simulink model "l1_lqr"  (R2025b)
settings: Solver=VariableStepAuto  StartTime=0.0  StopTime=10.0  RelTol=1e-3
undefined symbols (not defined in the file or in its folder): P
settings Model: Creator=eshikapathak  LastModifiedBy=eshikapathak

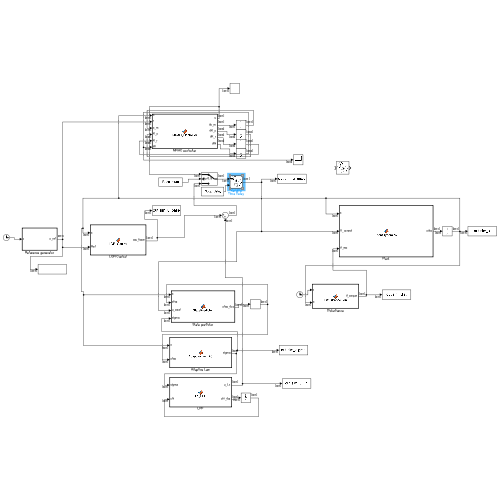
[thumbnail: Simulink's stored preview of the top-level diagram]
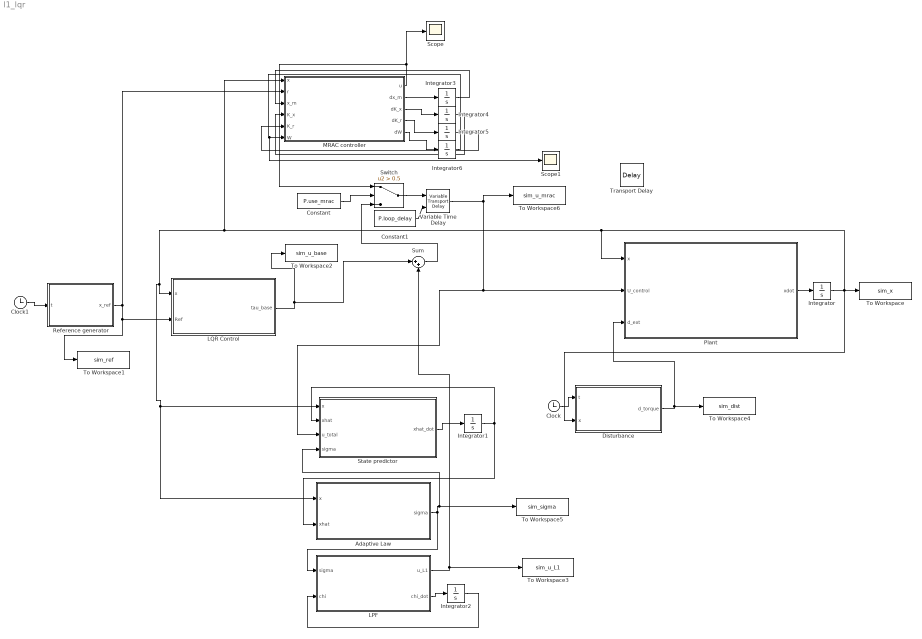
== system l1_lqr ==
  Adaptive Law : MATLAB Function  TreatAsAtomicUnit=on
  Clock : Clock
  Clock1 : Clock
  Constant : Constant  Value=P.use_mrac
  Constant1 : Constant  Value=P.loop_delay
  Disturbance : MATLAB Function  TreatAsAtomicUnit=on
  Integrator{,1..3} (4 alike) : Integrator
  Integrator4 : Integrator  InitialCondition=zeros(3,6)
  Integrator5 : Integrator  InitialCondition=zeros(3,6)
  Integrator6 : Integrator  InitialCondition=zeros(6,3)
  LPF : MATLAB Function  TreatAsAtomicUnit=on
  LQR Control : MATLAB Function  TreatAsAtomicUnit=on
  MRAC controller : MATLAB Function  TreatAsAtomicUnit=on
  Plant : MATLAB Function  TreatAsAtomicUnit=on
  Reference generator : MATLAB Function  TreatAsAtomicUnit=on
  Scope : Scope
      settings: ActiveDisplayYMinimum=-0.18899254495545503  ActiveDisplayYMaximum=0.88826024956797955
  Scope1 : Scope
      settings: ActiveDisplayYMinimum=-17.081145138179366  ActiveDisplayYMaximum=47.040865807014455
  State predictor : MATLAB Function  TreatAsAtomicUnit=on
  Sum : Sum  Inputs=|++
  Switch : Switch  Criteria=u2 > Threshold  Threshold=0.5  SaturateOnIntegerOverflow=off  InputSameDT=off
  To Workspace : ToWorkspace  VariableName=sim_x  SaveFormat=Timeseries  SampleTime=-1
  To Workspace1 : ToWorkspace  VariableName=sim_ref  SaveFormat=Timeseries  SampleTime=-1
  To Workspace2 : ToWorkspace  VariableName=sim_u_base  SaveFormat=Timeseries  SampleTime=-1
  To Workspace3 : ToWorkspace  VariableName=sim_u_L1  SaveFormat=Timeseries  SampleTime=-1
  To Workspace4 : ToWorkspace  VariableName=sim_dist  SaveFormat=Timeseries  SampleTime=-1
  To Workspace5 : ToWorkspace  VariableName=sim_sigma  SaveFormat=Timeseries  SampleTime=-1
  To Workspace6 : ToWorkspace  VariableName=sim_u_mrac  SaveFormat=Timeseries  SampleTime=-1
  Transport Delay : TransportDelay  DelayTime=P.loop_delay  BufferSize=10000000
  Variable Time Delay : VariableTransportDelay  MaximumDelay=10  MaximumPoints=1000000  ZeroDelay=on
  wires:
  Plant/1(xdot) -> Integrator/1
  Integrator/1 -> Disturbance/2(x), To Workspace/1, Plant/1(x), MRAC controller/1(x), LQR Control/1(x), Adaptive Law/1(x), State predictor/1(x)
  Reference generator/1(x_ref) -> LQR Control/2(Ref), To Workspace1/1, MRAC controller/2(r)
  Clock/1 -> Disturbance/1(t)
  Clock1/1 -> Reference generator/1(t)
  LQR Control/1(tau_base) -> To Workspace2/1, Sum/1
  LPF/1(u_L1) -> To Workspace3/1, Sum/2
  State predictor/1(xhat_dot) -> Integrator1/1
  Integrator1/1 -> Adaptive Law/2(xhat), State predictor/2(xhat)
  Adaptive Law/1(sigma) -> To Workspace5/1, State predictor/4(sigma), LPF/1(sigma)
  LPF/2(chi_dot) -> Integrator2/1
  Integrator2/1 -> LPF/2(chi)
  Variable Time Delay/1 -> To Workspace6/1, State predictor/3(u_total), Plant/2(U_control)
  Disturbance/1(d_torque) -> To Workspace4/1, Plant/3(d_ext)
  Switch/1 -> Variable Time Delay/1
  MRAC controller/2(dx_m) -> Integrator3/1
  MRAC controller/3(dK_x) -> Integrator4/1
  MRAC controller/4(dK_r) -> Integrator5/1
  Integrator3/1 -> MRAC controller/3(x_m)
  Integrator4/1 -> MRAC controller/4(K_x)
  Integrator5/1 -> MRAC controller/5(K_r)
  MRAC controller/1(u) -> Scope/1, Switch/1
  Sum/1 -> Switch/3
  Constant/1 -> Switch/2
  MRAC controller/5(dW) -> Integrator6/1
  Integrator6/1 -> Scope1/1, MRAC controller/6(W)
  Constant1/1 -> Variable Time Delay/2

== matlab function l1_lqr/LQR Control ==
  settings: sampleTime=P.Ts/100
  data: x input; tau_base output size=[3 1]; Ref input; P parameter
function tau_base = LQR_Control(x, Ref, P)
    % Standard State Feedback
    error = x - Ref;
    tau_base = -P.K * error;
end

== matlab function l1_lqr/Plant ==
  data: x input; xdot output size=[6 1]; U_control input; d_ext input; P parameter
function xdot = PlantDynamics(x, U_control, d_ext, P)
    % Unpack parameters
    Ix = P.Ix; Iy = P.Iy; Iz = P.Iz; L = P.L;
    
    % States
    % x = [phi, theta, psi, p, q, r]
    p = x(4); q = x(5); r = x(6);
    
    % Total Torque = Control Input + External Disturbance
    % U_control is [U2(Roll), U3(Pitch), U4(Yaw)] 
    % Inputs to this block are TORQUES.
    
    tau_phi   = L * U_control(1) + d_ext(1);
    tau_theta = L * U_control(2) + d_ext(2);
    tau_psi   =     U_control(3) + d_ext(3); 
    
    % Rotational Dynamics (Euler Equations)
    p_dot = q*r*(Iy - Iz)/Ix + (1/Ix) * tau_phi;
    q_dot = p*r*(Iz - Ix)/Iy + (1/Iy) * tau_theta;
    r_dot = p*q*(Ix - Iy)/Iz + (1/Iz) * tau_psi;
    
    % Kinematics 
    phi_dot   = p;
    theta_dot = q;
    psi_dot   = r;
    
    xdot = [phi_dot; theta_dot; psi_dot; p_dot; q_dot; r_dot];
end

== matlab function l1_lqr/State predictor ==
  data: x input; xhat_dot output size=[6 1]; xhat input; u_total input; sigma input; P parameter
% function xhat_dot = StatePredictor(x, xhat, u_total, sigma, P)
function xhat_dot = StatePredictor(x, xhat, u_total, sigma, P)
    % Unpack sigma into Matched (m) and Unmatched (um)
    sigma_m  = sigma(1:3);
    sigma_um = sigma(4:6);

    xt = xhat - x;

    % Predictor Dynamics
    % xhat_dot = A*xhat + Bm*(u + sigma_m) + Bum*sigma_um + Ae*xt
    xhat_dot = P.A_true * x ...
             + P.Bm * (u_total + sigma_m) ...
             + P.Bum * sigma_um ...
             + P.Ae * xt;
end


%%  Nonlinear State Predictor for L1 Adaptive Control
% function xhat_dot = StatePredictor(x, xhat, u_total, sigma, P)
%     % Nonlinear State Predictor for L1 Adaptive Control
%     % Dynamics: xhat_dot = f(x, u) + Bm*sigma_m + Bum*sigma_um + Ae*xt
% 
%     % 1. Unpack Parameters
%     Ix = P.Ix; Iy = P.Iy; Iz = P.Iz; L = P.L;
% 
%     % 2. Unpack Estimated States (from xhat, NOT x)
%     % xhat = [phi, theta, psi, p, q, r]
%     p = x(4); 
%     q = x(5); 
%     r = x(6);
% 
%     % 3. Unpack Control Inputs (Forces/Torque)
%     % u_total = [RollForce, PitchForce, YawTorque]
%     U_roll  = u_total(1);
%     U_pitch = u_total(2);
%     U_yaw   = u_total(3);
% 
%     % 4. Calculate Nominal Nonlinear Dynamics: f(xhat, u)
%     % Kinematics 
%     phi_dot   = p;
%     theta_dot = q;
%     psi_dot   = r;
% 
%     % Rotational Dynamics (Nonlinear Euler Equations)
%     % Note: We apply the same physics scaling (L/I) as the Plant
%     p_dot = ( (Iy - Iz) * q * r + L * U_roll  ) / Ix;
%     q_dot = ( (Iz - Ix) * p * r + L * U_pitch ) / Iy;
%     r_dot = ( (Ix - Iy) * p * q +     U_yaw   ) / Iz;
% 
%     f_x_u = [phi_dot; theta_dot; psi_dot; p_dot; q_dot; r_dot];
% 
%     % 5. Adaptive Augmentation
%     % sigma_m (Matched) affects accelerations
%     % sigma_um (Unmatched) affects kinematics
%     sigma_m  = sigma(1:3);
%     sigma_um = sigma(4:6);
% 
%     % Map Sigma to State Space
%     % P.Bm already contains the 1/J and L/J scaling for the matched uncertainty
%     adaptive_term = P.Bm * sigma_m + P.Bum * sigma_um;
% 
%     % 6. Error Dynamics Injection (Stabilizing term)
%     xt = xhat - x;
%     error_correction = P.Ae * xt;
% 
%     % 7. Final Predictor Derivative
%     xhat_dot = f_x_u + adaptive_term + error_correction;
% end

== matlab function l1_lqr/Adaptive Law ==
  settings: updateMethod=DISCRETE  sampleTime=P.Ts
  data: x input; sigma output size=[6 1]; xhat input; P parameter
function sigma = AdaptiveLaw_PC(x, xhat, P)
    % Define persistent variables to hold sigma for the interval
    % Note: Sampling property of this block is set to discrete with sample time as P.Ts
    persistent sigma_hold
    if isempty(sigma_hold)
        sigma_hold = zeros(6,1);
    end
    
    % Error
    xt = xhat - x;
    
    % Calculations (Closed Form Piecewise Constant)
    % Phi = Ae^-1 * (exp(Ae*Ts) - I)
    % We calculate this dynamically or pass it in. 
    % For efficiency, perform this only once or pass pre-calcs in P.
    
    Phi = P.Ae \ (expm(P.Ae*P.Ts) - eye(6));
    E   = expm(P.Ae*P.Ts);
    
    % z = Phi^-1 * exp(Ae*Ts) * xt(k)
    z = Phi \ (E * xt);
    
    % Bbar * sigma = -z
    % Bbar is square (6x6) because it is [Bm Bum]
    Bbar = [P.Bm, P.Bum];
    
    sigma_new = -(Bbar \ z);
    
    sigma = sigma_new;
end

== matlab function l1_lqr/LPF ==
  data: sigma input; u_L1 output size=[3 1]; chi input; chi_dot output size=[3 1]; P parameter
function [u_L1, chi_dot] = L1_LPF(sigma, chi, P)
    % 1. Extract Matched Uncertainty
    % The LPF only filters the matched component (first 3 elements)
    sigma_m = sigma(1:3);
    
    % 2. Filter Dynamics (State Space)
    % chi_dot = Alpf * chi + Blpf * sigma_m
    chi_dot = P.Alpf * chi + P.Blpf * sigma_m;
    
    % 3. Calculate Control Signal
    % u_L1 = - (Clpf * chi) 
    % We apply the negative sign here to cancel the disturbance.
    % (Dlpf is zero in this design, so we skip it)
    
    u_L1 = -(P.Clpf * chi);
end

== matlab function l1_lqr/Reference generator ==
  data: t input; x_ref output size=[6 1]; P parameter
function x_ref = ReferenceGen(t, P)
    % P.ref_type: 0 = Step, 1 = Sine
    
    ref_roll = 0;
    
    if P.ref_type == 0
        % --- STEP REFERENCE ---
        if t >= P.ref_start
            ref_roll = P.ref_amp;
        end
    else
        % --- SINE REFERENCE ---
        % Amplitude * sin(freq * t)
        % Using fixed 0.5 rad/s freq for testing
        ref_roll = P.ref_amp * sin(1.0 * t); 
    end
    
    % Output: [phi; theta; psi; p; q; r]
    x_ref = [ref_roll; 0; 0; 0; 0; 0];
end

== matlab function l1_lqr/Disturbance ==
  data: t input; x input; d_torque output size=[3 1]; P parameter
function d_torque = DisturbanceGen(t, x, P)
    % Generates disturbance torques (Nm) based on P.dist_type
    % Accepts state 'x' for state-dependent disturbances
    % P.dist_type: 
    %   0 = Single Sine
    %   1 = Sum of High Freq Sines
    %   2 = Triangle / Sawtooth
    %   3 = State-Dependent (Nonlinear)
    
    if isfield(P, 'dist_type')
        type = P.dist_type;
    else
        type = 0;
    end
    
    d_val = 0;

    if type == 0
        % Single Sine
        d_phi   = P.dist_amp(1) * sin(P.dist_freq(1) * t);
        d_theta = P.dist_amp(2) * sin(P.dist_freq(2) * t);
        d_psi   = P.dist_amp(3) * sin(P.dist_freq(3) * t);
        d_torque = [d_phi; d_theta; d_psi];
        return;
        
    elseif type == 1
        % Sum of Sines
        amp = P.dist_amp(1);
        d_val = 0.5 * amp * (sin(20*t) + sin(30*t) + sin(50*t));
        
    elseif type == 2
        % Triangle Wave
        freq = 2.0; amp = P.dist_amp(1);
        T = 2*pi/freq; norm_t = t/T;
        wave = 2 * abs(2 * (norm_t - floor(norm_t + 0.5))) - 1;
        d_val = amp * wave;
        
    elseif type == 3
        % --- STATE DEPENDENT (NONLINEAR) ---
        % d(x) = A * sin(3*phi) * p
        phi = x(1);
        p   = x(4);
        amp = P.dist_amp(1);
        
        d_val = amp * sin(3*phi) * p;
    end
    
    d_torque = [d_val; 0; 0]; 
end

== matlab function l1_lqr/MRAC controller ==
  data: x input; u output size=[3 1]; r input; x_m input size=[6 1]; K_x input; K_r input; W input; dx_m output; dK_x output size=[3 6]; dK_r output size=[3 6]; P parameter; dW output size=[6 3]
function [u, dx_m, dK_x, dK_r, dW] = MRAC_Controller(x, r, x_m, K_x, K_r, W, P)
    % --- 1. UNPACK PARAMETERS ---
    Am = P.MRAC.Am;
    Bm = P.MRAC.Bm;
    Gam_x = P.MRAC.Gam_x;
    Gam_r = P.MRAC.Gam_r;
    Gam_w = P.MRAC.Gam_w; 
    P_lyap = P.MRAC.P_lyap;
    B = P.Bm; 
    
    % Bounds for Projection (from P struct)
    th_x_max = P.MRAC.theta_x_max;
    th_r_max = P.MRAC.theta_r_max;
    th_w_max = P.MRAC.theta_w_max;
    
    % --- 2. BASIS FUNCTIONS (Phi) ---
    p = x(4); q = x(5); rr = x(6); 
    Phi = [tanh(q*rr); tanh(p*rr); tanh(p*q); tanh(p); tanh(q); tanh(rr)];
           
    % --- 3. DYNAMICS & ERROR ---
    dx_m = Am * x_m + Bm * r;
    e = x - x_m;
    
    % --- 4. ADAPTATION DRIVE ---
    % Common term: B' * P * e
    drive = B' * P_lyap * e; 
    
    % --- 5. NOMINAL ADAPTIVE LAWS ---
    dK_x_nom = Gam_x * drive * x'; 
    dK_r_nom = -Gam_r * drive * r'; 
    dW_nom   = Gam_w * Phi * drive'; % Note: dW is typically Gamma * Phi * e'PB
    % Dimension check: Phi(6x1) * drive'(1x3) = 6x3. W is 6x3. Correct.
    
    % --- 6. PROJECTION OPERATOR ---
    % Apply projection to keep parameters bounded
    dK_x = Projection(K_x, dK_x_nom, th_x_max);
    dK_r = Projection(K_r, dK_r_nom, th_r_max);
    dW   = Projection(W,   dW_nom,   th_w_max);
    
    % --- 7. CONTROL LAW ---
    % u = -K_x*x + K_r*r - W'*Phi
    u = -K_x * x + K_r * r - W' * Phi;
end

% --- LOCAL HELPER FUNCTION: PROJECTION ---
function dy_proj = Projection(theta, dy, theta_max)
    % Implements Convex Projection Operator 
    % theta: Current parameter value (matrix or vector)
    % dy:    Nominal update rate
    % theta_max: Maximum allowed Frobenius norm
    
    epsilon = 0.1; % Smoothness buffer width
    
    % 1. Calculate Norm squared
    n2 = sum(sum(theta.^2)); % Squared Frobenius Norm
    th_max2 = theta_max^2;
    
    % 2. Convex Function f(theta)
    f = (n2 - th_max2) / (epsilon * th_max2);
    
    % 3. Gradient of f w.r.t theta
    % grad_f = (2 / (epsilon * theta_max^2)) * theta
    % We only need the direction, so we use theta itself for dot product logic
    
    % Check condition: Are we outside bounds AND trying to grow further?
    % Dot product of Gradient and Update Direction:
    grad_dot_dy = sum(sum(theta .* dy)); 
    
    if (f >= 0) && (grad_dot_dy > 0)
        % ACTIVE PROJECTION
        % Subtract the component of dy that points "outward" (normal to boundary)
        
        % Simplified Smooth Projection Formula:
        % dy_proj = dy - ( (grad_f' * dy) / ||grad_f||^2 ) * grad_f * f(theta)
        
        % Calculating terms for matrices:
        grad_f = (2 / (epsilon * th_max2)) * theta;
        grad_norm2 = sum(sum(grad_f.^2));
        grad_dot_dy_val = sum(sum(grad_f .* dy));
        
        % Avoid divide by zero if theta is 0 (shouldn't happen at boundary)
        if grad_norm2 > 1e-10
            subtraction = (grad_f * grad_dot_dy_val / grad_norm2) * min(1, f);
            dy_proj = dy - subtraction;
        else
            dy_proj = dy;
        end
    else
        % NO PROJECTION (Inside bounds or moving inwards)
        dy_proj = dy;
    end
end
